simulink model "ESP32_FL_BB"  (R2023a)
settings: Solver=FixedStepAuto  StartTime=0.0  StopTime=inf  FixedStep=0.02  RelTol=1e-3  EnableMultiTasking=on
undefined symbols (not defined in the file): Discrete, Time
libraries: arduinolib x4, arduinosensorlib x2, ctrlSharedLib x2, simulink x2, simulink_extras x1
settings Model: ExtModeTrigDuration=2  Creator=j.acevedom  LastModifiedBy=j.acevedom
settings OptimizationCC: UseFloatMulNetSlope=on  DefaultUnderspecifiedDataType=single  EnhancedBackFolding=on  PassReuseOutputArgsAs=Individual arguments  ZeroExternalMemoryAtStartup=off  ZeroInternalMemoryAtStartup=off  MaxStackSize=64  OptimizeBlockOrder=speed  DifferentSizesBufferReuse=on  OptimizationCustomize=off  EfficientTunableParamExpr=on
settings DebuggingCC: ParameterTunabilityLossMsg=error
settings HardwareCC: ProdBitPerPointer=32  ProdBitPerSizeT=32  ProdBitPerPtrDiffT=32  ProdLargestAtomicInteger=Long  ProdLargestAtomicFloat=Double  ProdWordSize=32  ProdHWDeviceType=ARM Compatible->ARM Cortex  TargetLargestAtomicInteger=Long  TargetLargestAtomicFloat=Double  TargetIntDivRoundTo=Zero  TargetEndianess=LittleEndian  TargetHWDeviceType=ARM Compatible->ARM Cortex  UseEmbeddedCoderFeatures=off
settings SFSimCC: SimCustomCompilerFlags=CFLAGS+= -O3 -ffast-math -mfloat-abi=hard -mfpu=fpv4-sp-d16 CXXFLAGS+= -O3 -ffast-math -mfloat-abi=hard -mfpu=fpv4-sp-d16  MATLABDynamicMemAlloc=off
settings RTWCC: Description=Embedded Coder  SystemTargetFile=ert.tlc  HardwareBoard=ESP32-WROOM(Arduino Compatible)  TLCOptions="-aInlineSetEventsForThisBaseRateFcn=TLC_FALSE -aSuppressMultiTaskScheduler=TLC_FALSE  -aRateBasedStepFcn=0"  TemplateMakefile=ert_default_tmf  Toolchain=ESP32  BuildConfiguration=Faster Runs
settings CodeAppCC: ForceParamTrailComments=on  IgnoreCustomStorageClasses=off  OperatorAnnotations=on  SimulinkDataObjDesc=on  SFDataObjDesc=on  MangleLength=10  InsertBlockDesc=on
settings ERTTargetCC: SupportContinuousTime=on  SupportNonInlinedSFcns=on  SupportVariableSizeSignals=on  ExtModeTransport=3  ExtModeStaticAlloc=on  ExtModeAutomaticAllocSize=off  ExtModeStaticAllocSize=65536  ExtModeMexFile=ext_xcp  ExtModeIntrfLevel=Level2 - Open

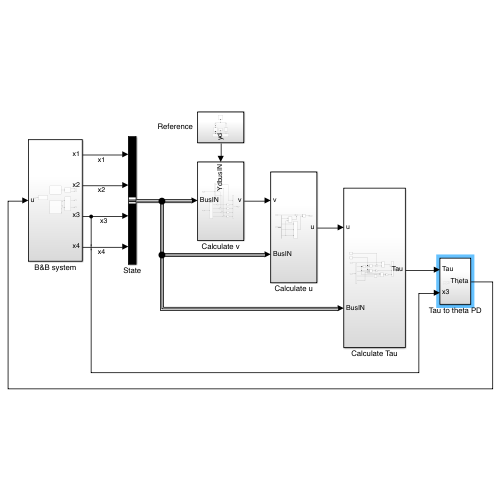
[thumbnail: Simulink's stored preview of the top-level diagram]
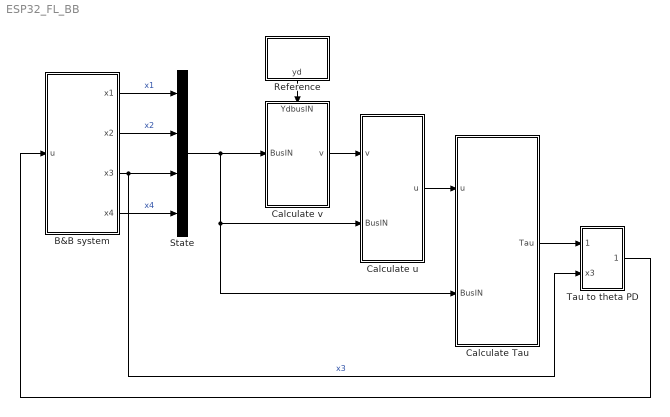
== system ESP32_FL_BB ==
  B&B system : Subsystem
  Calculate Tau : Subsystem
  Calculate u : Subsystem
  Calculate v : Subsystem
      settings: PortSchema="{\"entries\":[{\"content\":{\"sides\":[{\"content\":{\"connectorIds\":[\"In1\"]},\"type\":\"ConnectorPlacement.EquallySpacedRectSide\",\"uuid\":\"7c28e410-4806-4a94-8ccf-a14e347b0b8c\"},{\"content\":{\"connectorIds\":[\"Out1\"],\"side\":\"RIGHT\"},\"type\":\"ConnectorPlacement.EquallySpacedRectSide\",\"uuid\":\"f53d7206-bd2e-4f71-94df-5fcac3ff5314\"},{\"content\":{\"connectorIds\":[\"In2\"],\"side\":\"TOP\"},\"type\":\"ConnectorPlacement.EquallySpacedRectSide\",\"uuid\":\"6da5d2a6-a8d3-48a8-94f9-21942db04e1c\"}]},\"type\":\"ConnectorPlacement.EquallySpacedConnector\",\"uuid\":\"b4263dcd-b19e-4751-b906-56e55f698d2c\"}],\"packageUris\":[\"http://schema.mathworks.com/mf0/Connector/R2020b\"],\"version\":\"1.0\"}"
  Reference : Subsystem
  State : BusCreator  Inputs=4
  Tau to theta PD : Subsystem
  wires:
  Calculate u/1(u) -> Calculate Tau/1(u)
  State/1 -> Calculate Tau/2(BusIN), Calculate u/2(BusIN), Calculate v/1(BusIN)
  Calculate v/1(v) -> Calculate u/1(v)
  Calculate Tau/1(Tau) -> Tau to theta PD/1(Tau)
  B&B system/3(x3) -> State/3, Tau to theta PD/2(x3)  "x3"
  Tau to theta PD/1(Theta) -> B&B system/1(u)
  B&B system/1(x1) -> State/1  "x1"
  B&B system/2(x2) -> State/2  "x2"
  B&B system/4(x4) -> State/4  "x4"
  Reference/1(yd) -> Calculate v/2(YdbusIN)

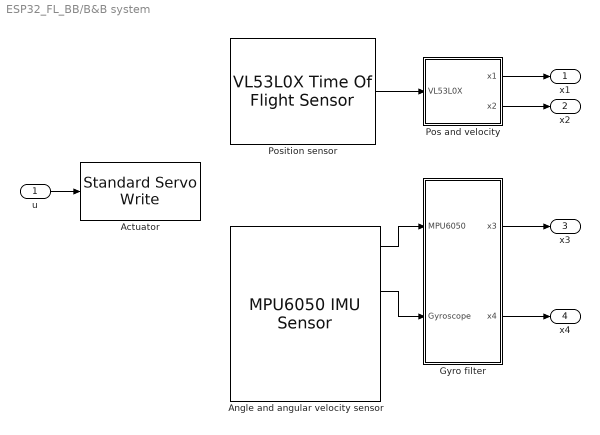
== system ESP32_FL_BB/B&B system ==
  u : Inport
  Actuator : arduinolib/Standard Servo Write  pinNumber=2  ServoIndex=0  blockPlatform=ESP3
  Angle and angular velocity sensor : arduinosensorlib/MPU6050 IMU Sensor  SlaveAddress=0x68  Accel=on  AngularRate=on  Temperature=on  Status=on  Timestamp=off  EulerAngles=off  Quat=off  AccelRange=2G  GyroRange=250 dps  DmpOdr=200 Hz  Dlpf=Accelerometer: 184Hz, Gyroscope: 188Hz  spf=1  SampleTime=-1  QueueSizeFactor=1
  Gyro filter : Subsystem
  Pos and velocity : Subsystem
  Position sensor : arduinosensorlib/VL53L0X Time Of Flight Sensor  I2CAddress=0x29  BitRate=1000000  RangingMode=High accuracy  SampleTime=-1
  x1 : Outport
  x2 : Outport  Port=2
  x3 : Outport  Port=3
  x4 : Outport  Port=4
  wires:
  Angle and angular velocity sensor/2 -> Gyro filter/2(Gyroscope)
  u/1 -> Actuator/1
  Pos and velocity/1(x1) -> x1/1
  Position sensor/1 -> Pos and velocity/1(VL53L0X)
  Angle and angular velocity sensor/1 -> Gyro filter/1(MPU6050)
  Gyro filter/1(x3) -> x3/1
  Gyro filter/2(x4) -> x4/1
  Pos and velocity/2(x2) -> x2/1

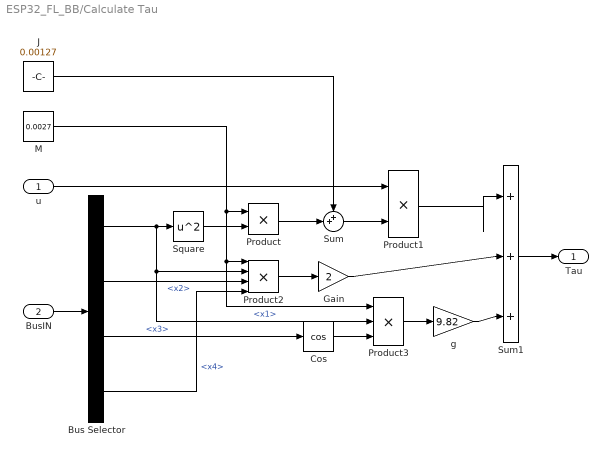
== system ESP32_FL_BB/Calculate Tau ==
  u : Inport
  BusIN : Inport  Port=2
  Bus Selector : BusSelector  OutputSignals=x1,x2,x3,x4
  Cos : Trigonometry  Operator=cos
  Gain : Gain  Gain=2
  J : Constant  Value=0.00127
  M : Constant  Value=0.0027
  Product : Product
  Product1 : Product
  Product2 : Product  Inputs=4
  Product3 : Product  Inputs=3
  Square : Math  Operator=square
  Sum : Sum  Inputs=++|
  Sum1 : Sum  Inputs=|+++
  g : Gain  Gain=9.82
  Tau : Outport
  wires:
  Square/1 -> Product/2
  M/1 -> Product2/1, Product3/1, Product/1
  Product/1 -> Sum/2
  J/1 -> Sum/1
  Sum/1 -> Product1/2
  u/1 -> Product1/1
  Bus Selector/4 -> Product2/4  "<x4>"
  Bus Selector/2 -> Product2/3  "<x2>"
  Bus Selector/1 -> Square/1, Product3/2, Product2/2  "<x1>"
  Product2/1 -> Gain/1
  Bus Selector/3 -> Cos/1  "<x3>"
  Gain/1 -> Sum1/2
  Product1/1 -> Sum1/1
  Sum1/1 -> Tau/1
  BusIN/1 -> Bus Selector/1
  Cos/1 -> Product3/3
  Product3/1 -> g/1
  g/1 -> Sum1/3

== system ESP32_FL_BB/Calculate u ==
  v : Inport
  BusIN : Inport  Port=2
  Divide : Product  Inputs=*/
  "State " : BusSelector  OutputSignals=x1,x2,x3,x4
  Sum : Sum  Inputs=|+-
  a calc : Subsystem
  b calc : Subsystem
  u : Outport
  wires:
  v/1 -> Sum/1
  Sum/1 -> Divide/1
  Divide/1 -> u/1
  "State "/4 -> b calc/2(x4), a calc/3(x4)  "<x4>"
  BusIN/1 -> "State "/1
  "State "/2 -> a calc/1(x2)  "<x2>"
  "State "/3 -> a calc/2(x3)  "<x3>"
  a calc/1(Out1) -> Divide/2
  "State "/1 -> b calc/1(x1)  "<x1>"
  b calc/1(b) -> Sum/2

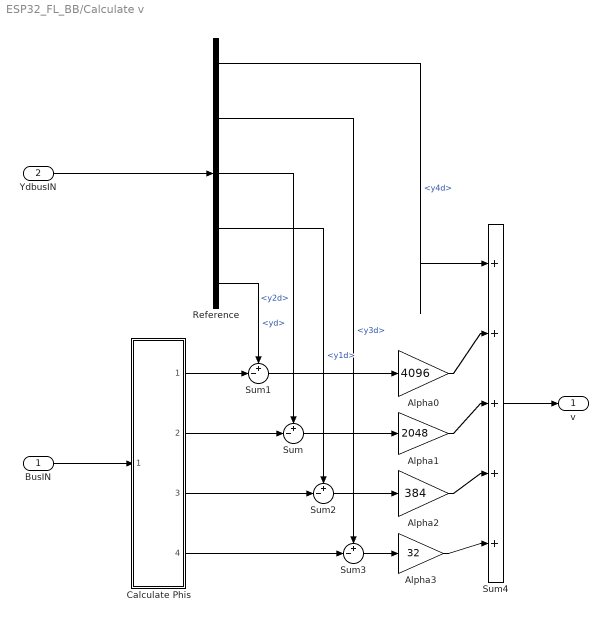
== system ESP32_FL_BB/Calculate v ==
  BusIN : Inport
  YdbusIN : Inport  Port=2
  Alpha0 : Gain  Gain=4096
  Alpha1 : Gain  Gain=2048
  Alpha2 : Gain  Gain=384
  Alpha3 : Gain  Gain=32
  Calculate Phis : Subsystem
  Reference : BusSelector  OutputSignals=y4d,y3d,y2d,y1d,yd
  Sum{,1..3} (4 alike) : Sum  Inputs=+-|
  Sum4 : Sum  Inputs=|+++++
  v : Outport
  wires:
  Sum2/1 -> Alpha2/1
  Sum3/1 -> Alpha3/1
  Reference/5 -> Sum1/1  "<yd>"
  Calculate Phis/1(Phi1) -> Sum1/2
  Reference/1 -> Sum4/1  "<y4d>"
  Reference/2 -> Sum3/1  "<y3d>"
  Reference/4 -> Sum2/1  "<y1d>"
  Alpha1/1 -> Sum4/3
  Alpha0/1 -> Sum4/2
  Alpha2/1 -> Sum4/4
  Sum/1 -> Alpha1/1
  Reference/3 -> Sum/1  "<y2d>"
  Alpha3/1 -> Sum4/5
  Calculate Phis/4(phi4) -> Sum3/2
  Sum1/1 -> Alpha0/1
  Calculate Phis/2(Phi2) -> Sum/2
  Calculate Phis/3(phi3) -> Sum2/2
  BusIN/1 -> Calculate Phis/1(BusIN)
  Sum4/1 -> v/1
  YdbusIN/1 -> Reference/1

== system ESP32_FL_BB/Reference ==
  Logic : Subsystem
  Switch1 : Switch  SaturateOnIntegerOverflow=off  InputSameDT=off
  potenciometer IN : arduinolib/Analog Input  pinNumber=6  ReadResultsOnly=off  ConversionTriggerSource=Software  ExternalTriggerType=uint32( 0 )  OutputDataType=uint16  EnableConversionCompleteNotify=off  EnableOuputStatus=off  SampleTime=-1  blockPlatform=arduino
  sine amp range : Gain  Gain=0.08/4095
  sine reference : Subsystem
  step range : Gain  Gain=0.4/4095  OutDataTypeStr=single
  step reference : Subsystem
  yd : Outport
  wires:
  step range/1 -> step reference/1(AIN)
  step reference/1(Step) -> Switch1/1
  Switch1/1 -> yd/1
  potenciometer IN/1 -> sine amp range/1, step range/1
  sine reference/1(Sine) -> Switch1/3
  Logic/1(Q) -> Switch1/2
  sine amp range/1 -> sine reference/1(AIN)

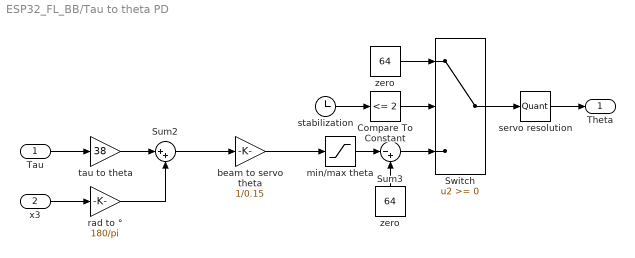
== system ESP32_FL_BB/Tau to theta PD ==
  Tau : Inport
  x3 : Inport  Port=2
  Compare To Constant : simulink/Logic and Bit Operations/Compare To Constant  relop=<=  const=2  OutDataTypeStr=boolean
  Sum2 : Sum  Inputs=|++
  Sum3 : Sum  Inputs=|-+
  Switch : Switch  SaturateOnIntegerOverflow=off  InputSameDT=off
  beam to servo theta : Gain  Gain=1/0.15
  min/max theta : Saturate  UpperLimit=60  LowerLimit=-60
  rad to ° : Gain  Gain=180/pi
  servo resolution : Quantizer  QuantizationInterval=1
  stabilization : Clock
  tau to theta : Gain  Gain=38
  zero : Constant  Value=64
  "zero " : Constant  Value=64
  Theta : Outport
  wires:
  x3/1 -> rad to °/1
  min/max theta/1 -> Sum3/1
  tau to theta/1 -> Sum2/1
  Sum3/1 -> Switch/3
  Compare To Constant/1 -> Switch/2
  stabilization/1 -> Compare To Constant/1
  "zero "/1 -> Sum3/2
  zero/1 -> Switch/1
  Sum2/1 -> beam to servo theta/1
  rad to °/1 -> Sum2/2
  Switch/1 -> servo resolution/1
  beam to servo theta/1 -> min/max theta/1
  Tau/1 -> tau to theta/1
  servo resolution/1 -> Theta/1

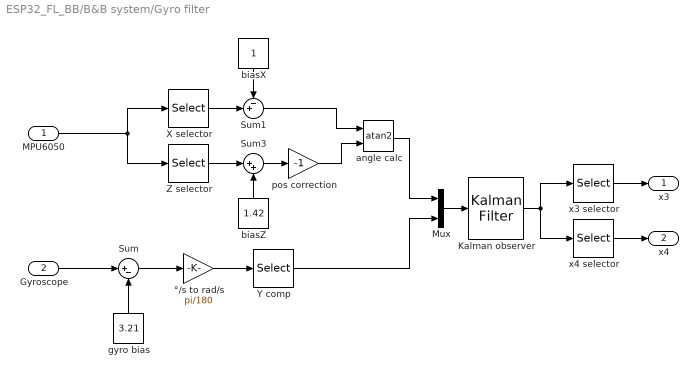
== system ESP32_FL_BB/B&B system/Gyro filter ==
  MPU6050 : Inport
  Gyroscope : Inport  Port=2
  Kalman observer : ctrlSharedLib/Kalman Filter  TimeDomain=Discrete-Time  UseCurrentEstimator=on  ModelSource=Individual A, B, C, D matrices  ModelSourceVariable=ss(0.95,1,1,0,1)  A=[1 0.02; 0 1]  B=1  C=[1 0; 0 1]  D=0  NumberOfStates=1  NumberOfInputs=1  NumberOfOutputs=1  InitialEstimateSource=Dialog  X0=[0; 0]  P0=10  UseK=off  UseGH=off  NumberOfProcessNoiseInputs=1  G=1  TimeInvariantG=on  H=0  TimeInvariantH=on  Q=[0.01 0; 0 0.001]  TimeInvariantQ=on  R=[1 0; 0 1]  TimeInvariantR=on  N=0  TimeInvariantN=on  AddInputPort=off  AddEnablePort=off  OutputEstimatedY=off  OutputP=off  Ts=0.02
  Mux : Mux  Inputs=2
  Sum : Sum  Inputs=|+-
  Sum1 : Sum  Inputs=-+|
  Sum3 : Sum  Inputs=|++
  X selector : Selector  NumberOfDimensions=2  InputPortWidth=3  IndexOptions=Index vector (dialog),Index vector (dialog)  Indices=1,1  OutputSizes=1,1
  Y comp : Selector  NumberOfDimensions=2  InputPortWidth=3  IndexOptions=Index vector (dialog),Index vector (dialog)  Indices=2,1  OutputSizes=1,1
  Z selector : Selector  NumberOfDimensions=2  InputPortWidth=3  IndexOptions=Index vector (dialog),Index vector (dialog)  Indices=3,1  OutputSizes=1,1
  angle calc : Trigonometry  Operator=atan2
  biasX : Constant
  biasZ : Constant  Value=1.42
  gyro bias : Constant  Value=3.21
  pos correction : Gain  Gain=-1
  x3 selector : Selector  NumberOfDimensions=2  InputPortWidth=3  IndexOptions=Index vector (dialog),Index vector (dialog)  Indices=1,1  OutputSizes=1,1
  x4 selector : Selector  NumberOfDimensions=2  InputPortWidth=3  IndexOptions=Index vector (dialog),Index vector (dialog)  Indices=2,1  OutputSizes=1,1
  °/s to rad/s : Gain  Gain=pi/180
  x3 : Outport
  x4 : Outport  Port=2
  wires:
  Gyroscope/1 -> Sum/1
  °/s to rad/s/1 -> Y comp/1
  gyro bias/1 -> Sum/2
  Sum/1 -> °/s to rad/s/1
  pos correction/1 -> angle calc/2
  Sum1/1 -> angle calc/1
  Sum3/1 -> pos correction/1
  MPU6050/1 -> X selector/1, Z selector/1
  biasX/1 -> Sum1/1
  X selector/1 -> Sum1/2
  biasZ/1 -> Sum3/2
  Z selector/1 -> Sum3/1
  Mux/1 -> Kalman observer/1
  Kalman observer/1 -> x3 selector/1, x4 selector/1
  x3 selector/1 -> x3/1
  x4 selector/1 -> x4/1
  angle calc/1 -> Mux/1
  Y comp/1 -> Mux/2

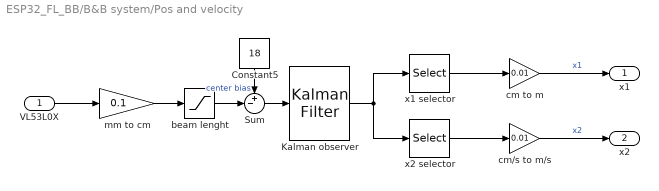
== system ESP32_FL_BB/B&B system/Pos and velocity ==
  VL53L0X : Inport
  Constant5 : Constant  Value=18
  Kalman observer : ctrlSharedLib/Kalman Filter  TimeDomain=Discrete-Time  UseCurrentEstimator=on  ModelSource=Individual A, B, C, D matrices  ModelSourceVariable=ss(0.95,1,1,0,1)  A=[1 0.02; 0 1]  B=1  C=[1 0]  D=0  NumberOfStates=1  NumberOfInputs=1  NumberOfOutputs=1  InitialEstimateSource=Dialog  X0=[0; 0]  P0=10  UseK=off  UseGH=off  NumberOfProcessNoiseInputs=1  G=1  TimeInvariantG=on  H=0  TimeInvariantH=on  Q=[0.0001 0; 0 0.1]  TimeInvariantQ=on  R=[0.05]  TimeInvariantR=on  N=0  TimeInvariantN=on  AddInputPort=off  AddEnablePort=off  OutputEstimatedY=off  OutputP=off  Ts=0.02
  Sum : Sum  Inputs=+-|
  beam lenght : Saturate  UpperLimit=40  LowerLimit=0
  cm to m : Gain  Gain=0.01
  cm/s to m/s : Gain  Gain=0.01
  mm to cm : Gain  Gain=0.1  OutDataTypeStr=single
  x1 selector : Selector  NumberOfDimensions=2  InputPortWidth=3  IndexOptions=Index vector (dialog),Index vector (dialog)  Indices=1,1  OutputSizes=1,1
  x2 selector : Selector  NumberOfDimensions=2  InputPortWidth=3  IndexOptions=Index vector (dialog),Index vector (dialog)  Indices=2,1  OutputSizes=1,1
  x1 : Outport
  x2 : Outport  Port=2
  wires:
  beam lenght/1 -> Sum/2
  Sum/1 -> Kalman observer/1
  mm to cm/1 -> beam lenght/1
  Kalman observer/1 -> x1 selector/1, x2 selector/1
  x1 selector/1 -> cm to m/1
  Constant5/1 -> Sum/1  "center bias"
  x2 selector/1 -> cm/s to m/s/1
  VL53L0X/1 -> mm to cm/1
  cm/s to m/s/1 -> x2/1  "x2"
  cm to m/1 -> x1/1  "x1"

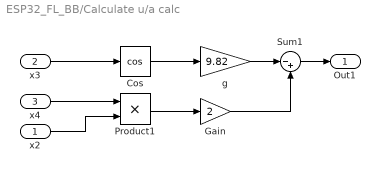
== system ESP32_FL_BB/Calculate u/a calc ==
  x2 : Inport
  x3 : Inport  Port=2
  x4 : Inport  Port=3
  Cos : Trigonometry  Operator=cos
  Gain : Gain  Gain=2
  Product1 : Product
  Sum1 : Sum  Inputs=|-+
  g : Gain  Gain=9.82
  Out1 : Outport
  wires:
  Product1/1 -> Gain/1
  Sum1/1 -> Out1/1
  Gain/1 -> Sum1/2
  Cos/1 -> g/1
  g/1 -> Sum1/1
  x3/1 -> Cos/1
  x4/1 -> Product1/1
  x2/1 -> Product1/2

== system ESP32_FL_BB/Calculate u/b calc ==
  x1 : Inport
  x4 : Inport  Port=2
  Math Function : Math  Operator=square
  Math Function1 : Math  Operator=square
  Product : Product
  b : Outport
  wires:
  Math Function/1 -> Math Function1/1
  Math Function1/1 -> Product/2
  x1/1 -> Product/1
  x4/1 -> Math Function/1
  Product/1 -> b/1

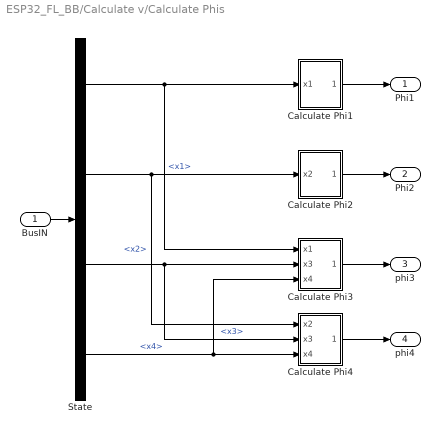
== system ESP32_FL_BB/Calculate v/Calculate Phis ==
  BusIN : Inport
  Calculate Phi1 : Subsystem
  Calculate Phi2 : Subsystem
  Calculate Phi3 : Subsystem
  Calculate Phi4 : Subsystem
  State : BusSelector  OutputSignals=x1,x2,x3,x4
  Phi1 : Outport
  Phi2 : Outport  Port=2
  phi3 : Outport  Port=3
  phi4 : Outport  Port=4
  wires:
  Calculate Phi1/1(Phi1) -> Phi1/1
  Calculate Phi3/1(phi3) -> phi3/1
  BusIN/1 -> State/1
  Calculate Phi4/1(phi4) -> phi4/1
  Calculate Phi2/1(Phi2) -> Phi2/1
  State/1 -> Calculate Phi3/1(x1), Calculate Phi1/1(x1)  "<x1>"
  State/2 -> Calculate Phi4/1(x2), Calculate Phi2/1(x2)  "<x2>"
  State/3 -> Calculate Phi4/2(x3), Calculate Phi3/2(x3)  "<x3>"
  State/4 -> Calculate Phi4/3(x4), Calculate Phi3/3(x4)  "<x4>"

== system ESP32_FL_BB/Reference/Logic ==
  Constant5 : Constant  OutDataTypeStr=boolean
  Constant8 : Constant  OutDataTypeStr=boolean
  J-K Flip-Flop : simulink_extras/Flip Flops/J-K Flip-Flop  initial_condition=0
  LED output : arduinolib/Digital Output  pinNumber=18  Direction=output  blockPlatform=arduino
  Rise detection : simulink/Logic and Bit Operations/Detect Rise Positive  vinit=0  OutDataTypeStr=boolean
  button in : arduinolib/Digital Input  pinNumber=5  mode=Default  Direction=input  SampleTime=0.02  blockPlatform=arduino
  Q : Outport
  wires:
  Rise detection/1 -> J-K Flip-Flop/2
  button in/1 -> Rise detection/1
  Constant8/1 -> J-K Flip-Flop/3
  Constant5/1 -> J-K Flip-Flop/1
  J-K Flip-Flop/1 -> Q/1, LED output/1

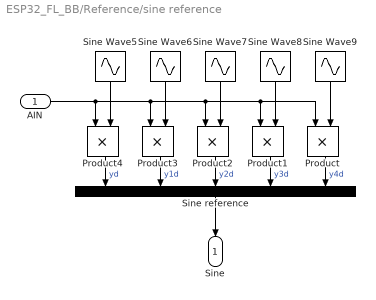
== system ESP32_FL_BB/Reference/sine reference ==
  AIN : Inport
  Product{,1..4} (5 alike) : Product
  Sine Wave5 : Sin  Frequency=pi  Phase=pi/2  SampleTime=0.02
  Sine Wave6 : Sin  Amplitude=-(1)*pi  Frequency=pi  SampleTime=0.02
  Sine Wave7 : Sin  Amplitude=-1*(pi)^2  Frequency=pi  Phase=pi/2  SampleTime=0.02
  Sine Wave8 : Sin  Amplitude=1*(pi)^3  Frequency=pi  SampleTime=0.02
  Sine Wave9 : Sin  Amplitude=1*(pi)^4  Frequency=pi  Phase=pi/2  SampleTime=0.02
  Sine reference : BusCreator  Inputs=5
  Sine : Outport
  wires:
  Sine Wave5/1 -> Product4/2
  Product/1 -> Sine reference/5  "y4d"
  Product2/1 -> Sine reference/3  "y2d"
  Sine Wave8/1 -> Product1/2
  Sine Wave9/1 -> Product/2
  Product4/1 -> Sine reference/1  "yd"
  Sine Wave7/1 -> Product2/2
  Sine Wave6/1 -> Product3/2
  Product3/1 -> Sine reference/2  "y1d"
  AIN/1 -> Product/1, Product1/1, Product2/1, Product3/1, Product4/1
  Product1/1 -> Sine reference/4  "y3d"
  Sine reference/1 -> Sine/1

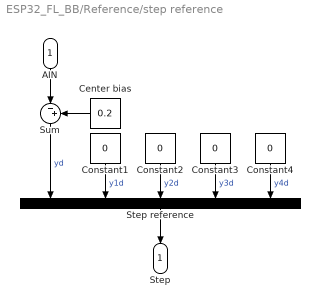
== system ESP32_FL_BB/Reference/step reference ==
  AIN : Inport
  Center bias : Constant  Value=0.2
  Constant{1..4} (4 alike) : Constant  Value=0
  Step reference : BusCreator  Inputs=5
  Sum : Sum  Inputs=|-+
  Step : Outport
  wires:
  Step reference/1 -> Step/1
  Constant2/1 -> Step reference/3  "y2d"
  Constant4/1 -> Step reference/5  "y4d"
  Constant1/1 -> Step reference/2  "y1d"
  AIN/1 -> Sum/1
  Constant3/1 -> Step reference/4  "y3d"
  Sum/1 -> Step reference/1  "yd"
  Center bias/1 -> Sum/2

== system ESP32_FL_BB/Calculate v/Calculate Phis/Calculate Phi1 ==
  x1 : Inport
  Phi1 : Outport
  wires:
  x1/1 -> Phi1/1

== system ESP32_FL_BB/Calculate v/Calculate Phis/Calculate Phi2 ==
  x2 : Inport
  Phi2 : Outport
  wires:
  x2/1 -> Phi2/1

== system ESP32_FL_BB/Calculate v/Calculate Phis/Calculate Phi3 ==
  x1 : Inport
  x3 : Inport  Port=2
  x4 : Inport  Port=3
  Math Function : Math  Operator=square
  Product : Product
  Sin : Trigonometry
  Sum : Sum  Inputs=-+|
  g : Gain  Gain=9.82
  phi3 : Outport
  wires:
  x4/1 -> Math Function/1
  x1/1 -> Product/1
  Math Function/1 -> Product/2
  x3/1 -> Sin/1
  Product/1 -> Sum/2
  g/1 -> Sum/1
  Sum/1 -> phi3/1
  Sin/1 -> g/1

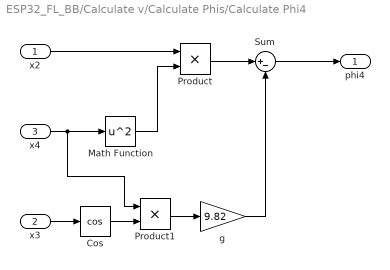
== system ESP32_FL_BB/Calculate v/Calculate Phis/Calculate Phi4 ==
  x2 : Inport
  x3 : Inport  Port=2
  x4 : Inport  Port=3
  Cos : Trigonometry  Operator=cos
  Math Function : Math  Operator=square
  Product : Product
  Product1 : Product
  Sum : Sum  Inputs=|+-
  g : Gain  Gain=9.82
  phi4 : Outport
  wires:
  x4/1 -> Product1/1, Math Function/1
  x2/1 -> Product/1
  Math Function/1 -> Product/2
  Product/1 -> Sum/1
  Sum/1 -> phi4/1
  x3/1 -> Cos/1
  Cos/1 -> Product1/2
  Product1/1 -> g/1
  g/1 -> Sum/2
